simulink model "powertrain_model"  (R2023a)
settings: Solver=VariableStepAuto  StartTime=0.0  StopTime=3557  RelTol=1e-3
values from neighbouring files (symbols this model uses):
  drivecycleData = readtable('extracted_data_filtered - Copy.csv')    [Drive_Cycle_Info.m]    (also in Old_Init.m = table2array(drivecycleData(:,2:5)); init.m = table2array(drivecycleData(:, 2:5)); loadDriveCycle-mar.m = table2array(drivecycleData(:,2:5)); loadDriveCycle.m = table2array(drivecycleData(:,2:5)))
  g = 9.8    [Old_Init.m]    (also in init.m; old_script.m)
  joules_to_kWh = 0.0000002778    (= 2.778e-07)    [Old_Init.m]    (also in init.m; old_script.m)
  lbs_to_kg = 0.45351    [Old_Init.m]    (also in init.m; old_script.m)
  meter_to_miles = 0.000621371    [Old_Init.m]    (also in init.m; old_script.m)
  mph_to_m_s = 0.44704    [Old_Init.m]    (also in init.m; old_script.m)
  optimal_gear_ratios = [index_columns,optimal_gear_ratios]    [Old_Init.m]    (also in init.m = [index_columns, optimal_gear_ratios]; old_script.m = [index_columns, optimal_gear_ratios])
  params = table2struct(vehicleData(strcmp(vehicleData.Make, vehicleName), :))    [Old_Init.m]    (also in VehicleParamsLoader.m = loadVehicleParams(vehicleType, obj.ExcelFilePath); getVehicleParams.m = table2struct(T(strcmp(T.Make, vehicleName), :)); init.m; loadParams.m = table2struct(T(strcmp(T.Make, targetMake), :)))
  SOC_init = 0.5    [Old_Init.m]    (also in init.m; loadVehicleParams.m; old_script.m)
undefined symbols (not defined in the file or in its folder): magnitude
libraries: BatteryEstimators x1
settings Model: Creator=cob_e  LastModifiedBy=Manuel

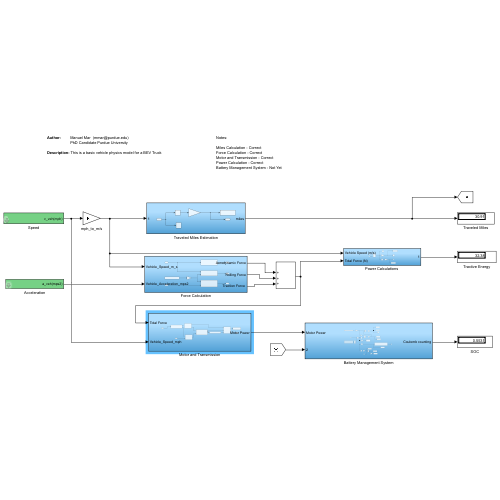
[thumbnail: Simulink's stored preview of the top-level diagram]
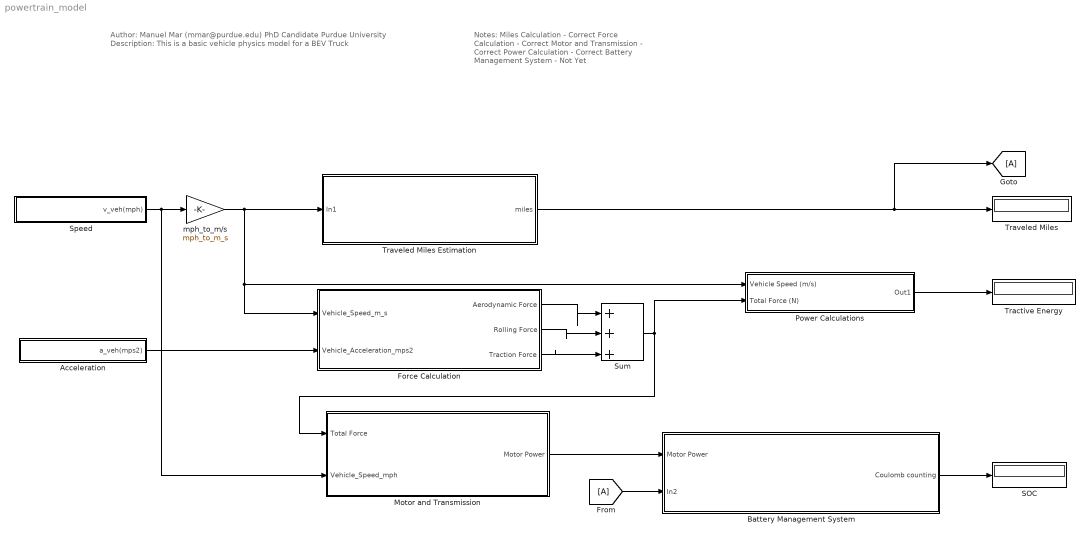
== system powertrain_model ==
  note: Notes:
      |
      | Miles Calculation - Correct
      | Force Calculation - Correct
      | Motor and Transmission - Correct
      | Power Calculation - Correct
      | Battery Management System - Not Yet
  note: Author: Manuel Mar (mmar@purdue.edu)
      | PhD Candidate Purdue University
      |
      | Description: This is a basic vehicle physics model for a BEV Truck
  Acceleration : Subsystem  mask{schedule=drivecycleData}
      mask prompts: schedule "drive schedule"
      mask init:
      | N=length(schedule(:,1))
  Battery Management System : Subsystem
  Force Calculation : Subsystem
  From : From
  Goto : Goto
  Motor and Transmission : Subsystem
  "Power Calculations " : Subsystem
  SOC : Display
  Speed : Subsystem  mask{schedule=drivecycleData}
      mask prompts: schedule "drive schedule"
      mask init:
      | N=length(schedule(:,1))
  Sum : Sum  Inputs=|+++
  Tractive Energy : Display
  Traveled Miles : Display
  Traveled Miles Estimation : Subsystem
  mph_to_m/s : Gain  Gain=mph_to_m_s
  wires:
  "Power Calculations "/1(Out1) -> Tractive Energy/1
  Sum/1 -> Motor and Transmission/1(Total Force), "Power Calculations "/2(Total Force (N))
  Speed/1(v_veh(mph)) -> Motor and Transmission/2(Vehicle_Speed_mph), mph_to_m/s/1
  Acceleration/1(a_veh(mps2)) -> Force Calculation/2(Vehicle_Acceleration_mps2)
  Force Calculation/1(Aerodynamic Force) -> Sum/1
  Force Calculation/2(Rolling Force) -> Sum/2
  Force Calculation/3("Traction Force ") -> Sum/3
  mph_to_m/s/1 -> "Power Calculations "/1(Vehicle Speed (m/s)), Force Calculation/1(Vehicle_Speed_m_s), Traveled Miles Estimation/1(In1)
  Motor and Transmission/1(Motor Power) -> Battery Management System/1(Motor Power)
  Battery Management System/1(Coulomb counting) -> SOC/1
  Traveled Miles Estimation/1(miles) -> Goto/1, Traveled Miles/1
  From/1 -> Battery Management System/2(In2)

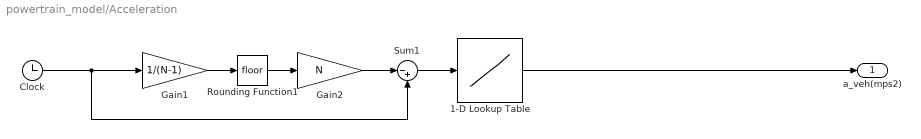
== system powertrain_model/Acceleration ==
  1-D Lookup Table : Lookup_n-D  NumberOfTableDimensions=1  BreakpointsForDimension1=schedule(:,1)  Table=schedule(:,4)  InternalRulePriority=Speed  RndMeth=Simplest
  Clock : Clock
  Gain1 : Gain  Gain=1/(N-1)
  Gain2 : Gain  Gain=N
  Rounding Function1 : Rounding
  Sum1 : Sum  Inputs=|-+
  a_veh(mps2) : Outport  VectorParamsAs1DForOutWhenUnconnected=off
  wires:
  Clock/1 -> Gain1/1, Sum1/2
  Sum1/1 -> 1-D Lookup Table/1
  Gain2/1 -> Sum1/1
  Rounding Function1/1 -> Gain2/1
  Gain1/1 -> Rounding Function1/1
  1-D Lookup Table/1 -> a_veh(mps2)/1

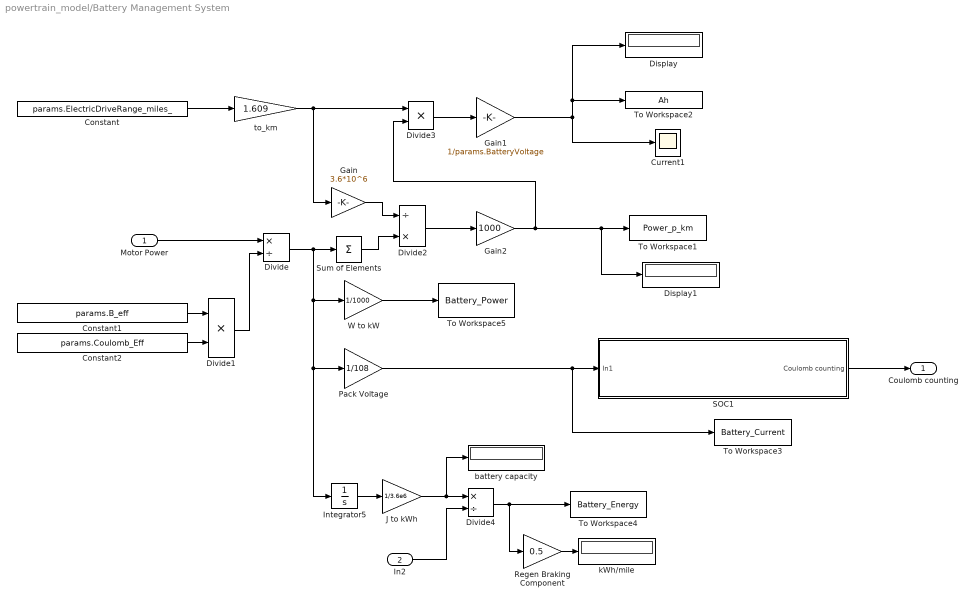
== system powertrain_model/Battery Management System ==
  Motor Power : Inport
  In2 : Inport  Port=2
  Constant : Constant  Value=params.ElectricDriveRange_miles_
  Constant1 : Constant  Value=params.B_eff
  Constant2 : Constant  Value=params.Coulomb_Eff
  Current1 : Scope
  Display : Display
  Display1 : Display
  Divide : Product  Inputs=*/
  Divide1 : Product  Inputs=**
  Divide2 : Product  Inputs=/*
  Divide3 : Product  Inputs=**
  Divide4 : Product  Inputs=*/
  Gain : Gain  Gain=3.6*10^6
  Gain1 : Gain  Gain=1/params.BatteryVoltage
  Gain2 : Gain  Gain=1000
  Integrator5 : Integrator
  J to kWh : Gain  Gain=1/3.6e6
  Pack Voltage : Gain  Gain=1/108
  Regen Braking Component : Gain  Gain=0.5
  SOC1 : Subsystem
  Sum of Elements : Sum  Inputs=+
  To Workspace1 : ToWorkspace  VariableName=Power_p_km  SaveFormat=Timeseries  SampleTime=-1
  To Workspace2 : ToWorkspace  VariableName=Ah  SaveFormat=Timeseries  SampleTime=-1
  To Workspace3 : ToWorkspace  VariableName=Battery_Current  SaveFormat=Timeseries  SampleTime=-1
  To Workspace4 : ToWorkspace  VariableName=Battery_Energy  SaveFormat=Timeseries  SampleTime=-1
  To Workspace5 : ToWorkspace  VariableName=Battery_Power  SaveFormat=Timeseries  SampleTime=-1
  W to kW : Gain  Gain=1/1000
  battery capacity : Display
  kWh/mile : Display
  to_km : Gain  Gain=1.609
  Coulomb counting : Outport
  wires:
  Divide/1 -> Pack Voltage/1, Integrator5/1, W to kW/1, Sum of Elements/1
  Integrator5/1 -> J to kWh/1
  to_km/1 -> Divide3/1, Gain/1
  SOC1/1(Coulomb counting) -> Coulomb counting/1
  Gain/1 -> Divide2/1
  Sum of Elements/1 -> Divide2/2
  Pack Voltage/1 -> To Workspace3/1, SOC1/1(In1)
  J to kWh/1 -> battery capacity/1, Divide4/1
  Constant1/1 -> Divide1/1
  Gain2/1 -> Divide3/2, Display1/1, To Workspace1/1
  Gain1/1 -> To Workspace2/1, Display/1, Current1/1
  W to kW/1 -> To Workspace5/1
  Divide4/1 -> Regen Braking Component/1, To Workspace4/1
  Constant2/1 -> Divide1/2
  Divide2/1 -> Gain2/1
  Divide1/1 -> Divide/2
  Divide3/1 -> Gain1/1
  Motor Power/1 -> Divide/1
  Constant/1 -> to_km/1
  In2/1 -> Divide4/2
  Regen Braking Component/1 -> kWh/mile/1

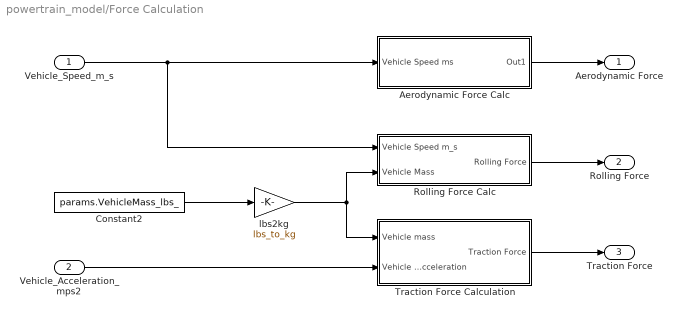
== system powertrain_model/Force Calculation ==
  Vehicle_Speed_m_s : Inport
  Vehicle_Acceleration_mps2 : Inport  Port=2
  Aerodynamic Force Calc : Subsystem
  Constant2 : Constant  Value=params.VehicleMass_lbs_
  Rolling Force Calc : Subsystem
  "Traction Force Calculation " : Subsystem
  lbs2kg : Gain  Gain=lbs_to_kg
  Aerodynamic Force : Outport
  Rolling Force : Outport  Port=2
  "Traction Force " : Outport  Port=3
  wires:
  Vehicle_Speed_m_s/1 -> Rolling Force Calc/1(Vehicle Speed m_s), Aerodynamic Force Calc/1(Vehicle Speed ms)
  Vehicle_Acceleration_mps2/1 -> "Traction Force Calculation "/2(Vehicle Acceleration)
  lbs2kg/1 -> "Traction Force Calculation "/1("Vehicle mass "), Rolling Force Calc/2(Vehicle Mass)
  "Traction Force Calculation "/1(Traction Force) -> "Traction Force "/1
  Rolling Force Calc/1(Rolling Force) -> Rolling Force/1
  Constant2/1 -> lbs2kg/1
  Aerodynamic Force Calc/1(Out1) -> Aerodynamic Force/1

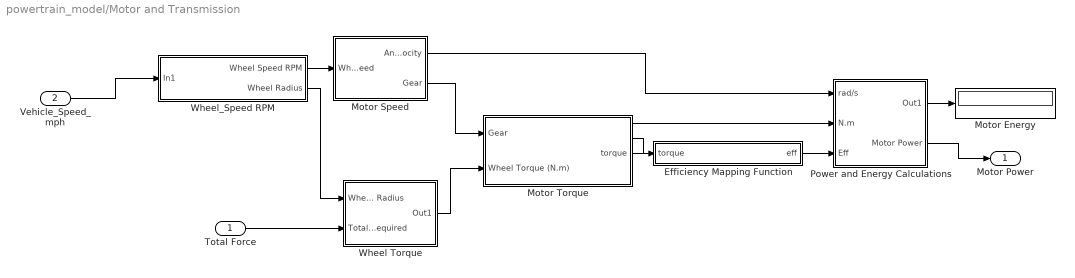
== system powertrain_model/Motor and Transmission ==
  Total Force : Inport
  Vehicle_Speed_mph : Inport  Port=2
  Efficiency Mapping Function : Subsystem
  Motor Energy : Display
  Motor Speed : Subsystem
  Motor Torque : Subsystem
  Power and Energy Calculations : Subsystem
  Wheel Torque : Subsystem
  Wheel_Speed RPM : Subsystem
  Motor Power : Outport
  wires:
  Total Force/1 -> Wheel Torque/2(Total Force Required)
  Motor Torque/1(torque) -> Efficiency Mapping Function/1(torque), Power and Energy Calculations/2(N.m)
  Vehicle_Speed_mph/1 -> Wheel_Speed RPM/1(In1)
  Power and Energy Calculations/1(Out1) -> Motor Energy/1
  Wheel_Speed RPM/2(Wheel Radius) -> Wheel Torque/1(Wheel Radius)
  Efficiency Mapping Function/1(eff) -> Power and Energy Calculations/3(Eff)
  Wheel Torque/1(Out1) -> Motor Torque/2(Wheel Torque (N.m))
  Motor Speed/1(Angular Velocity) -> Power and Energy Calculations/1(rad/s)
  Wheel_Speed RPM/1(Wheel Speed RPM) -> Motor Speed/1(Wheel Speed)
  Motor Speed/2(Gear) -> Motor Torque/1(Gear)
  Power and Energy Calculations/2(Motor Power) -> Motor Power/1

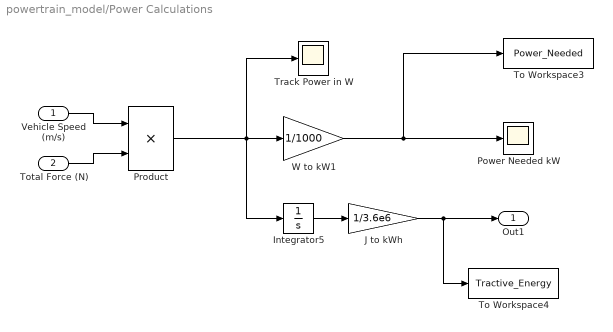
== system powertrain_model/Power Calculations  ==
  Vehicle Speed (m/s) : Inport
  Total Force (N) : Inport  Port=2
  Integrator5 : Integrator
  J to kWh : Gain  Gain=1/3.6e6
  Power Needed kW : Scope
  Product : Product
  To Workspace3 : ToWorkspace  VariableName=Power_Needed  SaveFormat=Timeseries  SampleTime=-1
  To Workspace4 : ToWorkspace  VariableName=Tractive_Energy  SaveFormat=Timeseries  SampleTime=-1
  Track Power in W : Scope
  W to kW1 : Gain  Gain=1/1000
  Out1 : Outport
  wires:
  Total Force (N)/1 -> Product/2
  J to kWh/1 -> Out1/1, To Workspace4/1
  Vehicle Speed (m/s)/1 -> Product/1
  Integrator5/1 -> J to kWh/1
  W to kW1/1 -> To Workspace3/1, Power Needed kW/1
  Product/1 -> W to kW1/1, Track Power in W/1, Integrator5/1

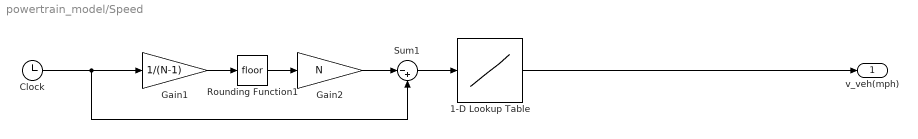
== system powertrain_model/Speed ==
  1-D Lookup Table : Lookup_n-D  NumberOfTableDimensions=1  BreakpointsForDimension1=schedule(:,1)  Table=schedule(:,3)  InternalRulePriority=Speed  RndMeth=Simplest
  Clock : Clock
  Gain1 : Gain  Gain=1/(N-1)
  Gain2 : Gain  Gain=N
  Rounding Function1 : Rounding
  Sum1 : Sum  Inputs=|-+
  v_veh(mph) : Outport  VectorParamsAs1DForOutWhenUnconnected=off
  wires:
  Clock/1 -> Gain1/1, Sum1/2
  Sum1/1 -> 1-D Lookup Table/1
  Gain2/1 -> Sum1/1
  Rounding Function1/1 -> Gain2/1
  Gain1/1 -> Rounding Function1/1
  1-D Lookup Table/1 -> v_veh(mph)/1

== system powertrain_model/Traveled Miles Estimation ==
  In1 : Inport
  Integrator4 : Integrator
  Scope : Scope
  To Workspace6 : ToWorkspace  VariableName=Miles_Traveled  SaveFormat=Timeseries  SampleTime=-1
  m_to_mi : Gain  Gain=meter_to_miles
  miles : Outport
  wires:
  In1/1 -> Scope/1, Integrator4/1
  m_to_mi/1 -> miles/1, To Workspace6/1  "miles"
  Integrator4/1 -> m_to_mi/1

== system powertrain_model/Battery Management System/SOC1 ==
  In1 : Inport
  Constant3 : Constant  Value=SOC_init
  Pack Voltage4 : Gain  Gain=1/(0.067*3600)
  SOC Estimator (Coulomb Counting) : BatteryEstimators/SOC Estimator (Coulomb Counting)  AH=27  Ts=1
      settings: LibrarySourceBlock=|
      | batt_sl_lib/Estimators/SOC Estimator
      | (Coulomb Counting)
  SOC1 : Scope
  To Workspace6 : ToWorkspace  VariableName=SOC  SaveFormat=Timeseries  SampleTime=-1
  Coulomb counting : Outport
  wires:
  Constant3/1 -> SOC Estimator (Coulomb Counting)/2
  SOC Estimator (Coulomb Counting)/1 -> To Workspace6/1, SOC1/1, Coulomb counting/1  "Coulomb counting"
  Pack Voltage4/1 -> SOC Estimator (Coulomb Counting)/1
  In1/1 -> Pack Voltage4/1

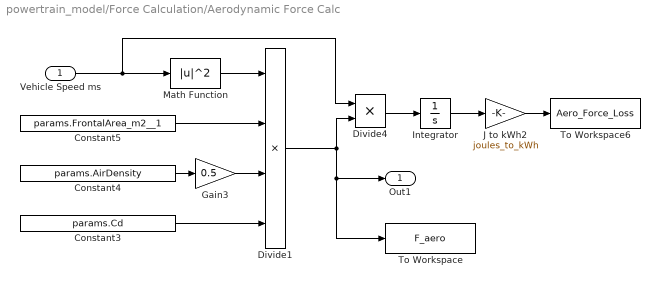
== system powertrain_model/Force Calculation/Aerodynamic Force Calc ==
  Vehicle Speed ms : Inport
  Constant3 : Constant  Value=params.Cd
  Constant4 : Constant  Value=params.AirDensity
  Constant5 : Constant  Value=params.FrontalArea_m2__1
  Divide1 : Product  Inputs=****
  Divide4 : Product  Inputs=**
  Gain3 : Gain  Gain=0.5
  Integrator : Integrator
  J to kWh2 : Gain  Gain=joules_to_kWh
  Math Function : Math  Operator=magnitude^2
  To Workspace : ToWorkspace  VariableName=F_aero  SaveFormat=Timeseries  SampleTime=-1
  To Workspace6 : ToWorkspace  VariableName=Aero_Force_Loss  SaveFormat=Timeseries  SampleTime=-1
  Out1 : Outport
  wires:
  Gain3/1 -> Divide1/3
  Divide4/1 -> Integrator/1
  Vehicle Speed ms/1 -> Divide4/1, Math Function/1
  Constant3/1 -> Divide1/4
  Constant5/1 -> Divide1/2
  Integrator/1 -> J to kWh2/1
  J to kWh2/1 -> To Workspace6/1
  Divide1/1 -> Divide4/2, To Workspace/1, Out1/1
  Constant4/1 -> Gain3/1
  Math Function/1 -> Divide1/1

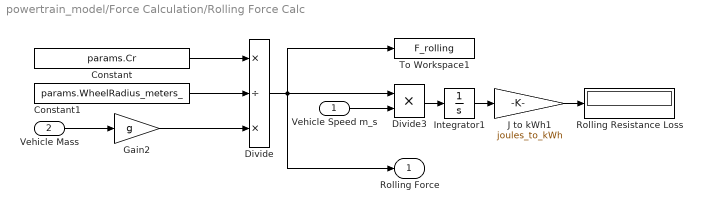
== system powertrain_model/Force Calculation/Rolling Force Calc ==
  Vehicle Speed m_s : Inport
  Vehicle Mass : Inport  Port=2
  Constant : Constant  Value=params.Cr
  Constant1 : Constant  Value=params.WheelRadius_meters_
  Divide : Product  Inputs=*/*
  Divide3 : Product  Inputs=**
  Gain2 : Gain  Gain=g
  Integrator1 : Integrator
  J to kWh1 : Gain  Gain=joules_to_kWh
  Rolling Resistance Loss : Display
  To Workspace1 : ToWorkspace  VariableName=F_rolling  SaveFormat=Timeseries  SampleTime=-1
  Rolling Force : Outport
  wires:
  Gain2/1 -> Divide/3
  Vehicle Speed m_s/1 -> Divide3/2
  Constant/1 -> Divide/1
  Integrator1/1 -> J to kWh1/1
  J to kWh1/1 -> Rolling Resistance Loss/1
  Vehicle Mass/1 -> Gain2/1
  Divide3/1 -> Integrator1/1
  Constant1/1 -> Divide/2
  Divide/1 -> To Workspace1/1, Rolling Force/1, Divide3/1

== system powertrain_model/Force Calculation/Traction Force Calculation  ==
  "Vehicle mass " : Inport
  Vehicle Acceleration : Inport  Port=2
  Divide2 : Product  Inputs=**
  To Workspace8 : ToWorkspace  VariableName=Traction_Force  SaveFormat=Timeseries  SampleTime=-1
  Traction Force : Outport
  wires:
  Divide2/1 -> To Workspace8/1, Traction Force/1
  Vehicle Acceleration/1 -> Divide2/2
  "Vehicle mass "/1 -> Divide2/1

== system powertrain_model/Motor and Transmission/Efficiency Mapping Function ==
  torque : Inport
  From Workspace : FromWorkspace  VariableName=N_m
  From Workspace1 : FromWorkspace  VariableName=Eff
  Gain : Gain  Gain=1/100
  MATLAB Function : MATLAB Function  TreatAsAtomicUnit=on
  Scope1 : Scope
  eff : Outport
  wires:
  From Workspace/1 -> MATLAB Function/2(N_m)
  From Workspace1/1 -> MATLAB Function/3(Eff)
  torque/1 -> MATLAB Function/1(torque)
  MATLAB Function/1(eff) -> Gain/1, Scope1/1
  Gain/1 -> eff/1

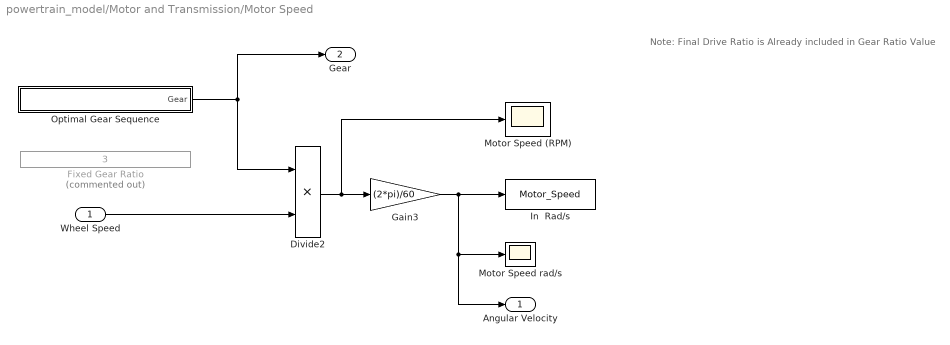
== system powertrain_model/Motor and Transmission/Motor Speed ==
  note: Note: Final Drive Ratio is Already included in Gear Ratio Value
  Wheel Speed : Inport
  Divide2 : Product  Inputs=**  RndMeth=Zero  SaturateOnIntegerOverflow=on
  Fixed Gear Ratio : Constant  Commented=on  Value=3
  Gain3 : Gain  Gain=(2*pi)/60
  In  Rad/s : ToWorkspace  VariableName=Motor_Speed  SaveFormat=Timeseries  SampleTime=-1
  Motor Speed (RPM) : Scope
  Motor Speed rad/s : Scope
  Optimal Gear Sequence : Subsystem  mask{schedule=optimal_gear_ratios}
      mask prompts: schedule "drive schedule"
      mask init:
      | N=length(schedule(:,1))
  Angular Velocity : Outport
  Gear : Outport  Port=2
  wires:
  Optimal Gear Sequence/1(Gear) -> Divide2/1, Gear/1
  Divide2/1 -> Gain3/1, Motor Speed (RPM)/1
  Gain3/1 -> Motor Speed rad/s/1, Angular Velocity/1, In  Rad/s/1
  Wheel Speed/1 -> Divide2/2

== system powertrain_model/Motor and Transmission/Motor Torque ==
  Gear : Inport
  Wheel Torque (N.m) : Inport  Port=2
  " " : Product  Inputs=/*
  Scope : Scope
  To Workspace : ToWorkspace  VariableName=Motor_Torque  SaveFormat=Timeseries  SampleTime=-1
  torque : Outport
  wires:
  " "/1 -> torque/1, Scope/1, To Workspace/1
  Gear/1 -> " "/1
  Wheel Torque (N.m)/1 -> " "/2

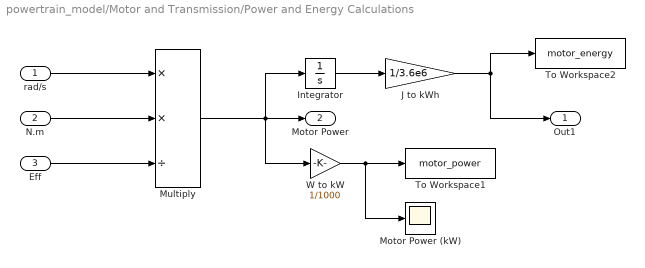
== system powertrain_model/Motor and Transmission/Power and Energy Calculations ==
  rad/s : Inport
  N.m : Inport  Port=2
  Eff : Inport  Port=3
  Integrator : Integrator
  J to kWh : Gain  Gain=1/3.6e6
  "Motor Power (kW) " : Scope
  Multiply : Product  Inputs=**/
  To Workspace1 : ToWorkspace  VariableName=motor_power  SaveFormat=Timeseries  SampleTime=-1
  To Workspace2 : ToWorkspace  VariableName=motor_energy  SaveFormat=Timeseries  SampleTime=-1
  W to kW : Gain  Gain=1/1000
  Out1 : Outport
  Motor Power : Outport  Port=2
  wires:
  Integrator/1 -> J to kWh/1
  Eff/1 -> Multiply/3
  Multiply/1 -> W to kW/1, Motor Power/1, Integrator/1
  W to kW/1 -> "Motor Power (kW) "/1, To Workspace1/1
  N.m/1 -> Multiply/2
  J to kWh/1 -> Out1/1, To Workspace2/1
  rad/s/1 -> Multiply/1

== system powertrain_model/Motor and Transmission/Wheel Torque ==
  Wheel Radius : Inport
  Total Force Required : Inport  Port=2
  Divide : Product  Inputs=**
  Wheel_Torque_Nm : Scope
  Out1 : Outport
  wires:
  Divide/1 -> Wheel_Torque_Nm/1, Out1/1
  Total Force Required/1 -> Divide/2
  Wheel Radius/1 -> Divide/1

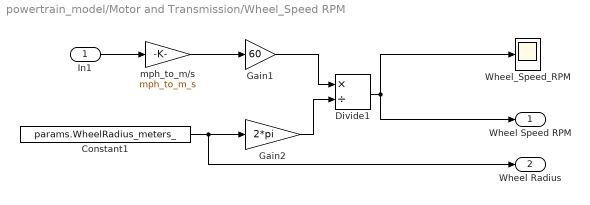
== system powertrain_model/Motor and Transmission/Wheel_Speed RPM ==
  In1 : Inport
  Constant1 : Constant  Value=params.WheelRadius_meters_
  Divide1 : Product  Inputs=*/
  Gain1 : Gain  Gain=60
  Gain2 : Gain  Gain=2*pi
  Wheel_Speed_RPM : Scope
  mph_to_m/s : Gain  Gain=mph_to_m_s
  Wheel Speed RPM : Outport
  Wheel Radius : Outport  Port=2
  wires:
  Constant1/1 -> Wheel Radius/1, Gain2/1
  Divide1/1 -> Wheel_Speed_RPM/1, Wheel Speed RPM/1
  Gain1/1 -> Divide1/1
  mph_to_m/s/1 -> Gain1/1
  Gain2/1 -> Divide1/2
  In1/1 -> mph_to_m/s/1

== system powertrain_model/Motor and Transmission/Motor Speed/Optimal Gear Sequence ==
  1-D Lookup Table : Lookup_n-D  NumberOfTableDimensions=1  BreakpointsForDimension1=schedule(:,1)  Table=schedule(:,2)  InternalRulePriority=Speed  RndMeth=Simplest
  Clock : Clock
  Gain1 : Gain  Gain=1/(N-1)
  Gain2 : Gain  Gain=N
  Rounding Function1 : Rounding
  Sum1 : Sum  Inputs=|-+
  Gear : Outport  VectorParamsAs1DForOutWhenUnconnected=off
  wires:
  Clock/1 -> Gain1/1, Sum1/2
  Sum1/1 -> 1-D Lookup Table/1
  Gain2/1 -> Sum1/1
  Rounding Function1/1 -> Gain2/1
  Gain1/1 -> Rounding Function1/1
  1-D Lookup Table/1 -> Gear/1

== matlab function powertrain_model/Motor and Transmission/Efficiency Mapping Function/MATLAB Function ==
  data: torque input; eff output; N_m input; Eff input
function eff = fcn(torque,N_m,Eff)
    % Define the same interpolation function here
    % N_m = [235.1 235 234.8 234.6 204.5 161.8 120.6];
    % Eff = [0 87.4 92.8 94.8 94.3 92.9 91.9];
    % 
    % Protect against out-of-range inputs
    if torque < min(N_m)
        torque = min(N_m);
    elseif torque > max(N_m)
        torque = max(N_m);
    end

    % Interpolation function for efficiency
    eff = interp1(N_m, Eff, torque, 'linear', 'extrap');
end
